simulink model "kessel_modell"  (R2024a)
settings: Solver=VariableStepAuto  StartTime=0.0  StopTime=2000  MaxStep=0.1  RelTol=1e-3
values from neighbouring files (symbols this model uses):
  KR = KR_LIST(i)    [kessel.m]    (also in kessel_loch.m = KR_list(i); kessel_loch_p.m; kessel_loch_pi.m = 0.01)
settings Model: Creator=janho  LastModifiedBy=janho

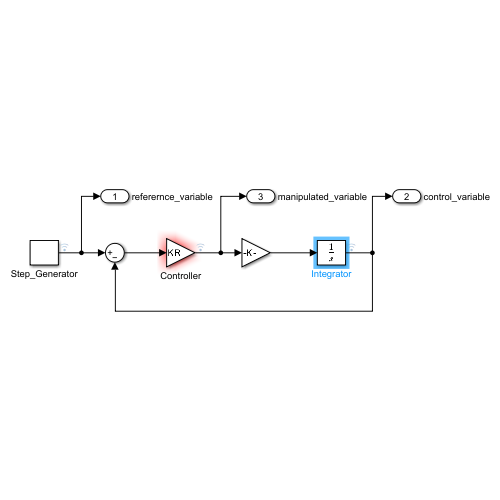
[thumbnail: Simulink's stored preview of the top-level diagram]
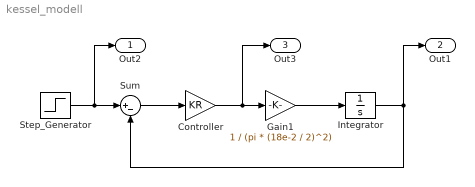
== system kessel_modell ==
  Controller : Gain  Gain=KR
  Gain1 : Gain  Gain=1 / (pi * (18e-2 / 2)^2)
  Integrator : Integrator
  Step_Generator : Step  Time=0  After=10e-2  SampleTime=0
  Sum : Sum  Inputs=|+-
  Out2 : Outport  SignalName=referernce_variable
  Out1 : Outport  Port=2  SignalName=control_variable
  Out3 : Outport  Port=3  SignalName=manipulated_variable
  wires:
  Integrator/1 -> Sum/2, Out1/1
  Sum/1 -> Controller/1
  Step_Generator/1 -> Out2/1, Sum/1
  Gain1/1 -> Integrator/1
  Controller/1 -> Out3/1, Gain1/1
